simulink subsystem "Triad"  (R2022b)
settings: Solver=VariableStepAuto  StartTime=0.0  StopTime=10.0  RelTol=1e-3
undefined symbols (not defined in the file or in its folder): sensors
libraries: sharedtransform x2
settings Model: Creator=robertopistonenascone  LastModifiedBy=robertopistonenascone

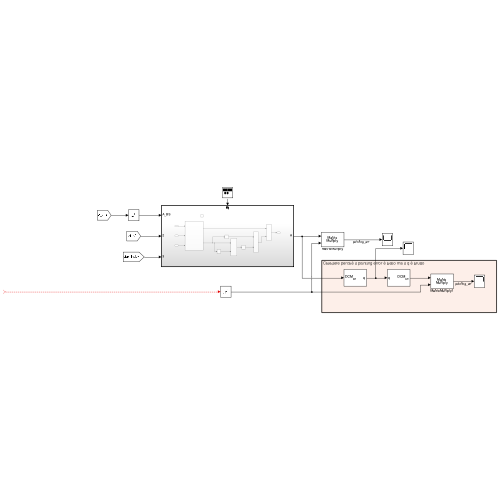
[thumbnail: Simulink's stored preview of the top-level diagram]
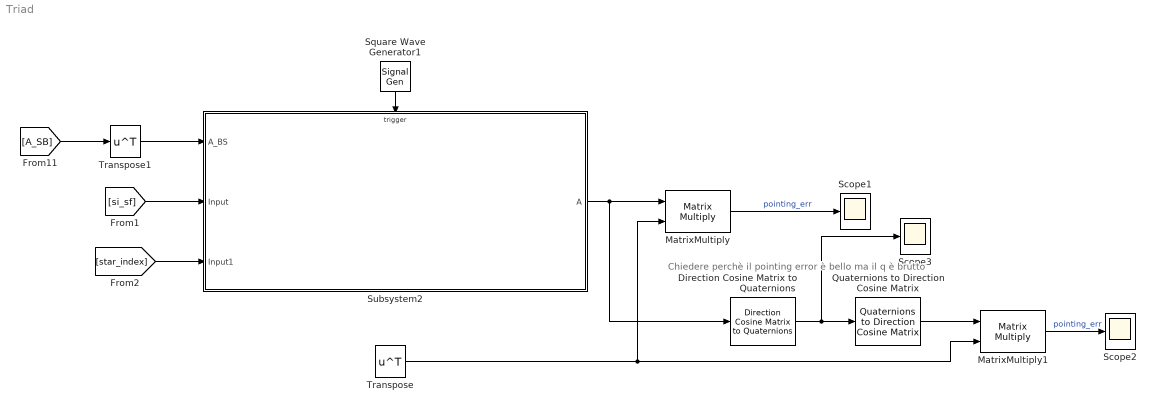
== system Triad ==
  note: Chiedere perchè il pointing error è bello ma il q è brutto
  Direction Cosine Matrix to Quaternions : sharedtransform/Direction Cosine Matrix  to Quaternions  aMode=0  action=None  tolerance=eps(2)
      settings: LibrarySourceBlock=|
      | aerolibtransform2/Direction Cosine Matrix
      | to Quaternions
  MatrixMultiply : Product  Multiplication=Matrix(*)
  MatrixMultiply1 : Product  Multiplication=Matrix(*)
  Quaternions to Direction Cosine Matrix : sharedtransform/Quaternions to  Direction Cosine Matrix  aMode=aMode
      settings: LibrarySourceBlock=|
      | aerolibtransform2/Quaternions to
      | Direction Cosine Matrix
  Scope1 : Scope
  Scope2 : Scope
  Scope3 : Scope
  Square Wave Generator1 : SignalGenerator  WaveForm=square  Frequency=sensors.star.frequency/2
  Subsystem2 : Subsystem
  Transpose : Math  Operator=transpose
  Transpose1 : Math  Operator=transpose
  wires:
  MatrixMultiply/1 -> Scope1/1  "pointing_err"
  Subsystem2/1(A) -> Direction Cosine Matrix to Quaternions/1, MatrixMultiply/1
  [A_SB] -> Transpose1/1
  Transpose1/1 -> Subsystem2/1(A_BS)
  Transpose/1 -> MatrixMultiply1/2, MatrixMultiply/2
  [si_sf] -> Subsystem2/2(Input)
  MatrixMultiply1/1 -> Scope2/1  "pointing_err"
  Direction Cosine Matrix to Quaternions/1 -> Scope3/1, Quaternions to Direction Cosine Matrix/1
  Square Wave Generator1/1 -> Subsystem2/Trigger
  [star_index] -> Subsystem2/3(Input1)
  Quaternions to Direction Cosine Matrix/1 -> MatrixMultiply1/1
  ? -> Transpose/1

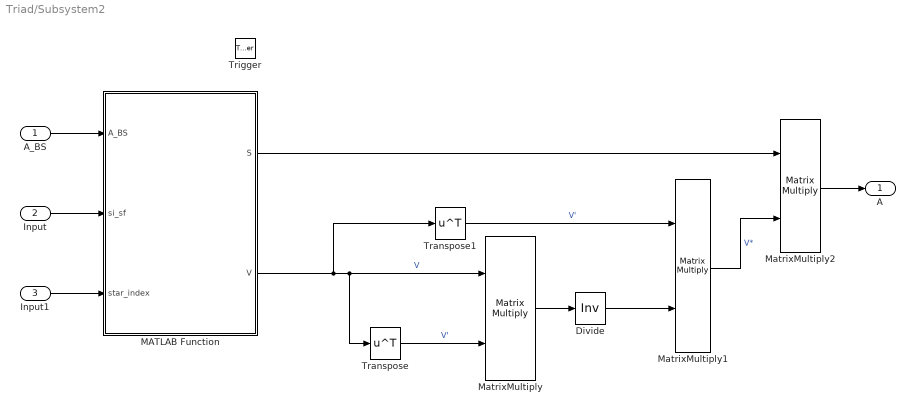
== system Triad/Subsystem2 ==
  A_BS : Inport
  Input : Inport  Port=2
  Input1 : Inport  Port=3
  Trigger : TriggerPort  TriggerType=either  VariantControl=(inherit)  PortDimensions=1
  Divide : Product  Inputs=/  Multiplication=Matrix(*)
  MATLAB Function : MATLAB Function  TreatAsAtomicUnit=on
  MatrixMultiply : Product  Multiplication=Matrix(*)
  MatrixMultiply1 : Product  Multiplication=Matrix(*)
  MatrixMultiply2 : Product  Multiplication=Matrix(*)
  Transpose : Math  Operator=transpose
  Transpose1 : Math  Operator=transpose
  A : Outport
  wires:
  Input1/1 -> MATLAB Function/3(star_index)
  Input/1 -> MATLAB Function/2(si_sf)
  A_BS/1 -> MATLAB Function/1(A_BS)
  MATLAB Function/2(V) -> Transpose1/1, Transpose/1, MatrixMultiply/1  "V"
  Transpose/1 -> MatrixMultiply/2  "V'"
  MatrixMultiply/1 -> Divide/1
  Divide/1 -> MatrixMultiply1/2
  Transpose1/1 -> MatrixMultiply1/1  "V'"
  MatrixMultiply1/1 -> MatrixMultiply2/2  "V*"
  MatrixMultiply2/1 -> A/1
  MATLAB Function/1(S) -> MatrixMultiply2/1

== matlab function Triad/Subsystem2/MATLAB Function ==
  data: S output; A_BS input; si_sf input; V output; star_index input; catalogue parameter
function [S, V] = triad(A_BS, si_sf, star_index, catalogue)

B = zeros(3, 3);
V = zeros(3, length(star_index));
S = zeros(3, length(star_index));

% vector of real star position
for k = 1:length(star_index)
    V(:, k) = (catalogue(star_index(k), (1:3)))';

    % rotation from sensor to body frame
    S(:, k) = A_BS*si_sf(k, :)';


end
